simulink model "NlinCloop"  (R2021a)
settings: Solver=VariableStepAuto  StartTime=0.0  StopTime=100  MaxStep=0.01  RelTol=1e-3
values from neighbouring files (symbols this model uses):
  g = 9.8    [Linearmodel.m]
  J = diag([2.7,3.3,5.4])    [Linearmodel.m]
  Jinv = J^-1    [Linearmodel.m]
  m = 0.254    [Linearmodel.m]
settings Model: Creator=Sirius  LastModifiedBy=Sirius

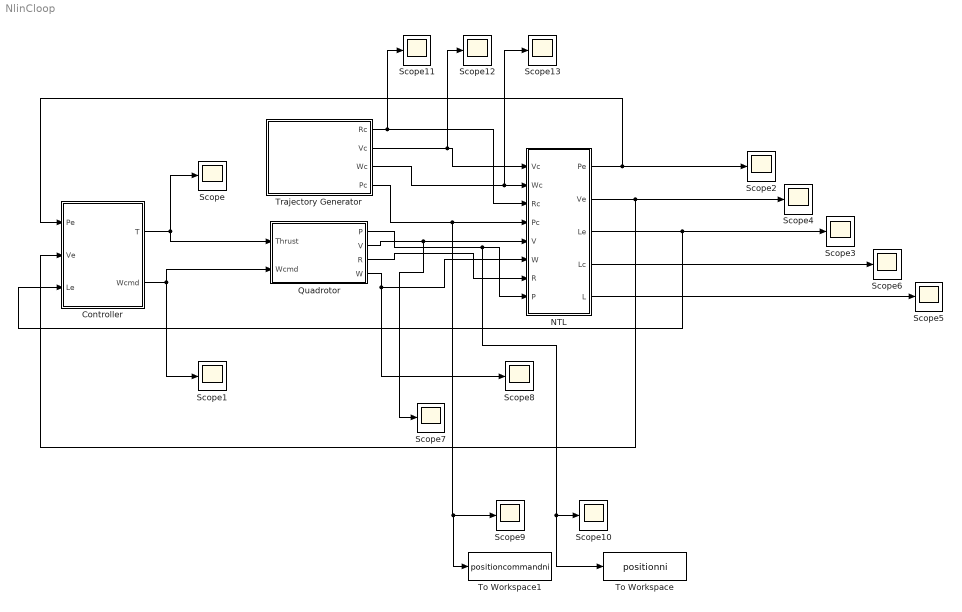
== system NlinCloop ==
  Controller : MATLAB Function  TreatAsAtomicUnit=on
  NTL : MATLAB Function  TreatAsAtomicUnit=on
  Quadrotor : Subsystem
  Scope{,1..13} (14 alike) : Scope
  To Workspace : ToWorkspace  VariableName=positionni  SaveFormat=Timeseries  SampleTime=-1
  To Workspace1 : ToWorkspace  VariableName=positioncommandni  SaveFormat=Timeseries  SampleTime=-1
  Trajectory Generator : Subsystem
  wires:
  Controller/1(T) -> Scope/1, Quadrotor/1(Thrust)
  Controller/2(Wcmd) -> Quadrotor/2(Wcmd), Scope1/1
  Trajectory Generator/2(Vc) -> Scope12/1, NTL/1(Vc)
  Trajectory Generator/3(Wc) -> Scope13/1, NTL/2(Wc)
  Trajectory Generator/1(Rc) -> Scope11/1, NTL/3(Rc)
  Trajectory Generator/4(Pc) -> To Workspace1/1, Scope9/1, NTL/4(Pc)
  NTL/5(L) -> Scope5/1
  NTL/4(Lc) -> Scope6/1
  NTL/3(Le) -> Controller/3(Le), Scope3/1
  NTL/2(Ve) -> Controller/2(Ve), Scope4/1
  NTL/1(Pe) -> Controller/1(Pe), Scope2/1
  Quadrotor/4(W) -> Scope8/1, NTL/6(W)
  Quadrotor/1(P) -> To Workspace/1, Scope10/1, NTL/8(P)
  Quadrotor/2(V) -> Scope7/1, NTL/5(V)
  Quadrotor/3(R) -> NTL/7(R)

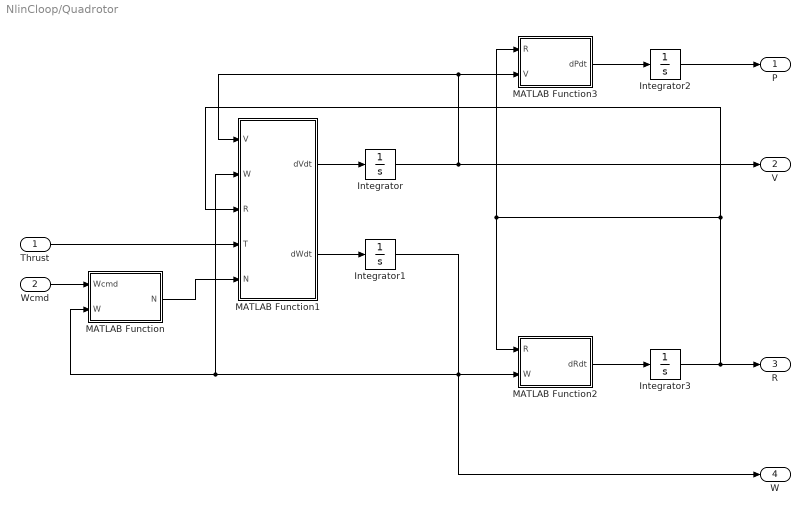
== system NlinCloop/Quadrotor ==
  Thrust : Inport
  Wcmd : Inport  Port=2
  Integrator : Integrator  InitialCondition=[0;0;0]
  Integrator1 : Integrator  InitialCondition=[0;0;0]
  Integrator2 : Integrator  InitialCondition=[0;1;0]
  Integrator3 : Integrator  InitialCondition=eye(3)
  MATLAB Function : MATLAB Function  TreatAsAtomicUnit=on
  MATLAB Function1 : MATLAB Function  TreatAsAtomicUnit=on
  MATLAB Function2 : MATLAB Function  TreatAsAtomicUnit=on
  MATLAB Function3 : MATLAB Function  TreatAsAtomicUnit=on
  P : Outport
  V : Outport  Port=2
  R : Outport  Port=3
  W : Outport  Port=4
  wires:
  MATLAB Function2/1(dRdt) -> Integrator3/1
  Wcmd/1 -> MATLAB Function/1(Wcmd)
  MATLAB Function1/1(dVdt) -> Integrator/1
  Thrust/1 -> MATLAB Function1/4(T)
  MATLAB Function1/2(dWdt) -> Integrator1/1
  MATLAB Function/1(N) -> MATLAB Function1/5(N)
  MATLAB Function3/1(dPdt) -> Integrator2/1
  Integrator/1 -> V/1, MATLAB Function1/1(V), MATLAB Function3/2(V)
  Integrator3/1 -> MATLAB Function1/3(R), MATLAB Function3/1(R), MATLAB Function2/1(R), R/1
  Integrator1/1 -> MATLAB Function1/2(W), MATLAB Function/2(W), W/1, MATLAB Function2/2(W)
  Integrator2/1 -> P/1

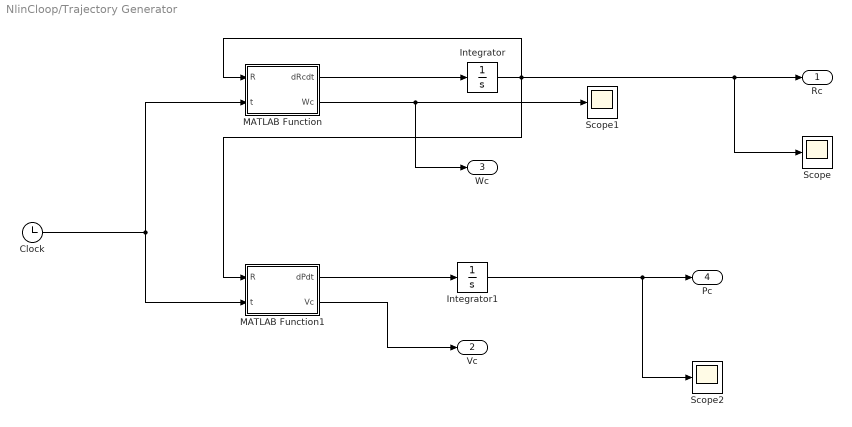
== system NlinCloop/Trajectory Generator ==
  Clock : Clock
  Integrator : Integrator  InitialCondition=eye(3)
  Integrator1 : Integrator  InitialCondition=[0;0;0]
  MATLAB Function : MATLAB Function  TreatAsAtomicUnit=on
  MATLAB Function1 : MATLAB Function  TreatAsAtomicUnit=on
  Scope : Scope
  Scope1 : Scope
  Scope2 : Scope
  Rc : Outport
  Vc : Outport  Port=2
  Wc : Outport  Port=3
  Pc : Outport  Port=4
  wires:
  MATLAB Function1/1(dPdt) -> Integrator1/1
  Integrator1/1 -> Scope2/1, Pc/1
  Integrator/1 -> MATLAB Function1/1(R), MATLAB Function/1(R), Scope/1, Rc/1
  MATLAB Function/2(Wc) -> Wc/1, Scope1/1
  MATLAB Function1/2(Vc) -> Vc/1
  Clock/1 -> MATLAB Function/2(t), MATLAB Function1/2(t)
  MATLAB Function/1(dRcdt) -> Integrator/1

== matlab function NlinCloop/Trajectory Generator/MATLAB Function ==
  data: R input; dRcdt output; t input; Wc output
function [dRcdt,Wc] =dRdt(R,t)

Wc=[0;0;0];
if((t>=19.5)&&(t<=20.5))
    Wc=[0;0;pi/2];
end
if((t>=39.5)&&(t<=40.5))
    Wc=[0;0;pi/2];
end
if((t>=59.5)&&(t<=60.5))
    Wc=[0;0;pi/2];
end
dRcdt=R*Skew(Wc);
end

== matlab function NlinCloop/Controller ==
  data: Pe input; T output; Ve input; Le input; Wcmd output; K parameter
function [T,Wcmd]=Controller(Pe,Ve,Le,K)
x=[Pe;Ve;Le];
u=-K*x;
T=u(1);
Wcmd=u(2:4);
end

== matlab function NlinCloop/Trajectory Generator/MATLAB Function1 ==
  data: R input; dPdt output; t input; Vc output
function [dPdt,Vc] = dPdt(R,t)
Vc=[0.5;0;0];
dPdt=R*Vc;
end

== matlab function NlinCloop/Quadrotor/MATLAB Function ==
  data: Wcmd input; N output; W input
function N = Wcontorl(Wcmd,W)
N=1000*(Wcmd-W);
end

== matlab function NlinCloop/Quadrotor/MATLAB Function1 ==
  data: V input; dVdt output; W input; R input; T input; N input; dWdt output; Jinv parameter; m parameter; g parameter; J parameter
function [dVdt,dWdt]=QDyanamics(V,W,R,T,N,Jinv, m, g, J)
Windforce = [0.5;0.5;0];% 0.5N along X and Y 
dVdt=-Skew(W)*V+1/m*([0;0;-T]+R'*[0;0;m*g]+Windforce);
dWdt=-Jinv*Skew(W)*J*W+Jinv*N;
end

== matlab function NlinCloop/Quadrotor/MATLAB Function2 ==
  data: R input; dRdt output; W input
function dRdt=dRdt(R,W)
dRdt=R*Skew(W);
end

== matlab function NlinCloop/Quadrotor/MATLAB Function3 ==
  data: R input; dPdt output; V input
function dPdt=dPdt(R,V)
dPdt=R*V;
end

== matlab function NlinCloop/NTL ==
  data: Vc input; Pe output; Wc input; Rc input; Pc input; V input; W input; R input; P input; Ve output; Le output; Lc output; L output
function [Pe,Ve,Le,Lc,L] = NLT(Vc,Wc,Rc,Pc,V,W,R,P)
Rc2b=R'*Rc;
Ve=V-Vc;
Pe=R'*(P-Pc);
Re=Rc'*R;
L=Rmat2PRY(R)*180/pi;
Lc=Rmat2PRY(Rc)*180/pi;
Le=Rmat2PRY(Re);
end
